simulink model "Model_v1"  (R2016b)
settings: Solver=VariableStepAuto  StartTime=0.0  StopTime=1.5  MaxStep=0.01  RelTol=1e-3
InitFcn:
  | start
values from neighbouring files (symbols this model uses):
  Psi0 = pi/12    (= 0.261799387799)    [start_config.m]
  Psi_d0 = 0    [start_config.m]
  Theta_d0 = 0    [start_config.m]
undefined symbols (not defined in the file or in its folder): A, B, K, Umax
libraries: simulink_extras x3
settings Model: PauseTimes=1  SnapshotBufferSize=8000  Creator=danii  LastModifiedBy=danii
settings SolverCC: ZeroCrossAlgorithm=Adaptive
settings ConfigComp: PSAutoStubLUT=on

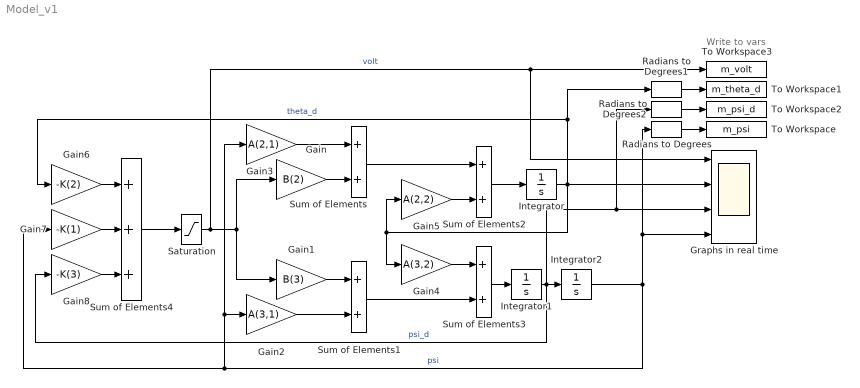
== system Model_v1 ==
  note: Write to vars
  Gain : Gain  Gain=B(2)
  Gain1 : Gain  Gain=B(3)
  Gain2 : Gain  Gain=A(3,1)
  Gain3 : Gain  Gain=A(2,1)
  Gain4 : Gain  Gain=A(3,2)
  Gain5 : Gain  Gain=A(2,2)
  Gain6 : Gain  Gain=-K(2)
  Gain7 : Gain  Gain=-K(1)
  Gain8 : Gain  Gain=-K(3)
  Graphs in real time : Scope  NumInputPorts=4
  Integrator : Integrator  InitialCondition=Theta_d0
  Integrator1 : Integrator  InitialCondition=Psi_d0
  Integrator2 : Integrator  InitialCondition=Psi0
  Radians to Degrees : simulink_extras/Transformations/Radians to Degrees
  Radians to Degrees1 : simulink_extras/Transformations/Radians to Degrees
  Radians to Degrees2 : simulink_extras/Transformations/Radians to Degrees
  Saturation : Saturate  UpperLimit=Umax  LowerLimit=-Umax
  Sum of Elements{,1..3} (4 alike) : Sum  Inputs=2
  Sum of Elements4 : Sum  Inputs=3
  To Workspace : ToWorkspace  VariableName=m_psi  SampleTime=-1
  To Workspace1 : ToWorkspace  VariableName=m_theta_d  SampleTime=-1
  To Workspace2 : ToWorkspace  VariableName=m_psi_d  SampleTime=-1
  To Workspace3 : ToWorkspace  VariableName=m_volt  SampleTime=-1
  wires:
  Saturation/1 -> Gain1/1, Gain/1, Graphs in real time/1, To Workspace3/1  "volt"
  Gain/1 -> Sum of Elements/2
  Gain1/1 -> Sum of Elements1/1
  Gain2/1 -> Sum of Elements1/2
  Gain3/1 -> Sum of Elements/1
  Sum of Elements/1 -> Sum of Elements2/1
  Sum of Elements1/1 -> Sum of Elements3/2
  Gain5/1 -> Sum of Elements2/2
  Gain4/1 -> Sum of Elements3/1
  Sum of Elements2/1 -> Integrator/1
  Sum of Elements3/1 -> Integrator1/1
  Integrator/1 -> Gain4/1, Gain5/1, Graphs in real time/2, Gain6/1, Radians to Degrees1/1  "theta_d"
  Integrator1/1 -> Integrator2/1, Gain8/1, Radians to Degrees2/1, Graphs in real time/3  "psi_d"
  Sum of Elements4/1 -> Saturation/1
  Gain7/1 -> Sum of Elements4/2
  Gain8/1 -> Sum of Elements4/3
  Radians to Degrees/1 -> To Workspace/1
  Radians to Degrees2/1 -> To Workspace2/1
  Radians to Degrees1/1 -> To Workspace1/1
  Integrator2/1 -> Gain7/1, Gain3/1, Gain2/1, Radians to Degrees/1, Graphs in real time/4  "psi"
  Gain6/1 -> Sum of Elements4/1
